simulink model "pid_model"  (Simulink 7.0)
settings: Solver=ode3  StartTime=0.0  StopTime=15  FixedStep=0.1  MaxStep=0.001  RelTol=1e-3
PreLoadFcn:
  | K = 12
undefined symbols (not defined in the file): Kf, mass, maxF
settings Model: Creator=nein  LastModifiedBy=nein

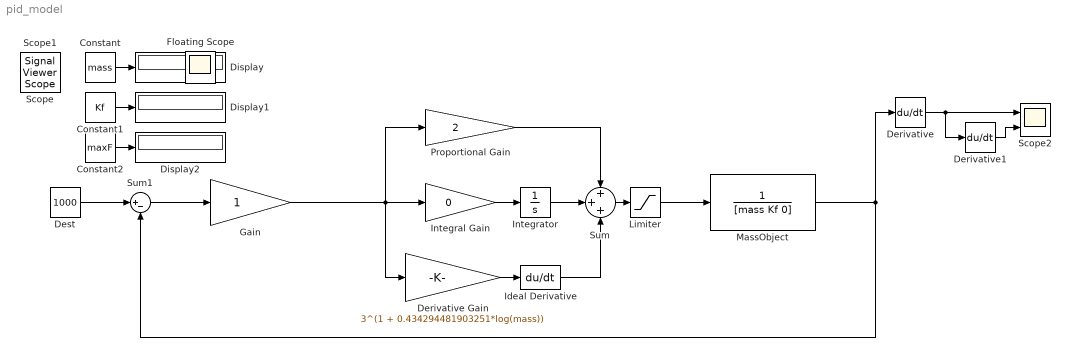
== system pid_model ==
  Constant : Constant  Value=mass  OutDataType=sfix(16)  OutScaling=2^0
  Constant1 : Constant  Value=Kf  OutDataType=sfix(16)  OutScaling=2^0
  Constant2 : Constant  Value=maxF  OutDataType=sfix(16)  OutScaling=2^0
  Derivative : Derivative
  Derivative Gain : Gain  Gain=3^(1 + 0.434294481903251*log(mass))  ParameterDataType=sfix(16)  ParameterScaling=2^0  OutDataType=sfix(16)  OutScaling=2^0  SaturateOnIntegerOverflow=on
  Derivative1 : Derivative
  Dest : Constant  Value=1000  OutDataType=sfix(16)  OutScaling=2^0
  Display : Display
  Display1 : Display
  Display2 : Display
  Gain : Gain  ParameterDataType=sfix(16)  ParameterScaling=2^0  OutDataType=sfix(16)  OutScaling=2^0
  Ideal Derivative : Derivative
  Integral Gain : Gain  Gain=0  ParameterDataType=sfix(16)  ParameterScaling=2^0  OutDataType=sfix(16)  OutScaling=2^0  SaturateOnIntegerOverflow=on
  Integrator : Integrator
  Limiter : Saturate  UpperLimit=maxF  LowerLimit=-maxF  OutDataType=sfix(16)  OutScaling=2^0
  MassObject : TransferFcn  Denominator=[mass Kf 0]
  Proportional Gain : Gain  Gain=2  ParameterDataType=sfix(16)  ParameterScaling=2^0  OutDataType=sfix(16)  OutScaling=2^0
  Scope2 : Scope  NumInputPorts=2
      settings: TimeRange=15  YMin=-50~-150  YMax=350~150
  Sum : Sum  Inputs=+++  OutDataType=sfix(16)  OutScaling=2^0  SaturateOnIntegerOverflow=on  InputSameDT=on
  Sum1 : Sum  Inputs=|+-  OutDataType=sfix(16)  OutScaling=2^0
  Floating Scope : Scope
      settings: Floating=on
  Scope : SignalViewerScope  IOType=viewer  RefreshTime=0.035000
  Scope1 : SignalViewerScope  IOType=viewer  RefreshTime=0.035000
      settings: TimeRange=15  YMin=-200  YMax=1200
  wires:
  Sum1/1 -> Gain/1
  MassObject/1 -> Sum1/2, Derivative/1
  Dest/1 -> Sum1/1
  Gain/1 -> Derivative Gain/1, Integral Gain/1, Proportional Gain/1
  Constant/1 -> Display/1
  Constant1/1 -> Display1/1
  Limiter/1 -> MassObject/1
  Constant2/1 -> Display2/1
  Sum/1 -> Limiter/1
  Proportional Gain/1 -> Sum/1
  Derivative Gain/1 -> Ideal Derivative/1
  Ideal Derivative/1 -> Sum/3
  Integrator/1 -> Sum/2
  Integral Gain/1 -> Integrator/1
  Derivative/1 -> Derivative1/1, Scope2/1
  Derivative1/1 -> Scope2/2
